simulink model "AERO560_HW1B_ThaparGagandeep"  (R2022b)
settings: Solver=VariableStepAuto  StartTime=0.0  StopTime=200.0  RelTol=1e-3
settings Model: Creator=gagandeepthapar  LastModifiedBy=gagandeepthapar

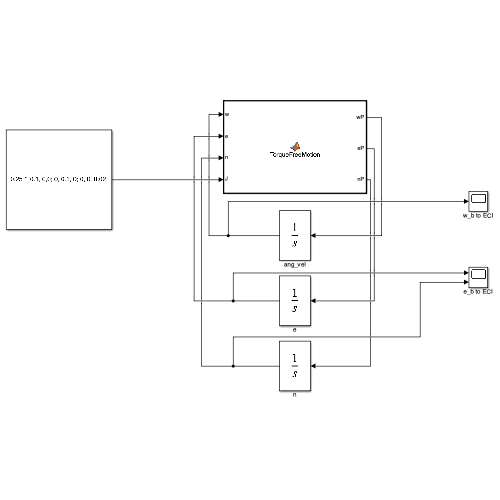
[thumbnail: Simulink's stored preview of the top-level diagram]
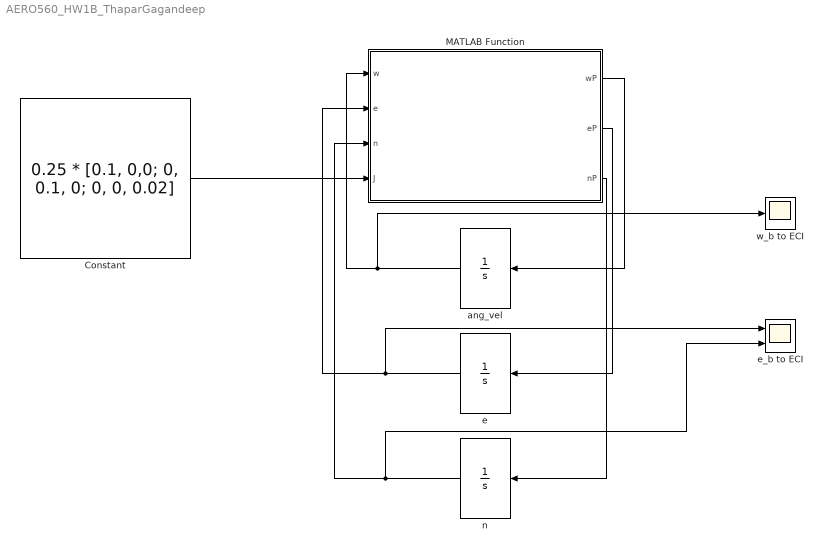
== system AERO560_HW1B_ThaparGagandeep ==
  Constant : Constant  Value=0.25 * [0.1, 0,0; 0, 0.1, 0; 0, 0, 0.02]
  MATLAB Function : MATLAB Function  TreatAsAtomicUnit=on
  ang_vel : Integrator  InitialCondition=[0.1; 0.1; 0.1]  ContinuousStateAttributes='ang_vel'
  e : Integrator  InitialCondition=[0;0;0]  ContinuousStateAttributes='e'
  e_b to ECI : Scope  NumInputPorts=2
  n : Integrator  InitialCondition=[1]  ContinuousStateAttributes='n'
  w_b to ECI : Scope
  wires:
  Constant/1 -> MATLAB Function/4(J)
  MATLAB Function/1(wP) -> ang_vel/1
  MATLAB Function/2(eP) -> e/1
  MATLAB Function/3(nP) -> n/1
  ang_vel/1 -> w_b to ECI/1, MATLAB Function/1(w)
  e/1 -> e_b to ECI/1, MATLAB Function/2(e)
  n/1 -> e_b to ECI/2, MATLAB Function/3(n)

== matlab function AERO560_HW1B_ThaparGagandeep/MATLAB Function ==
  data: w input; wP output; e input; n input; J input; eP output; nP output
function [wP, eP, nP] = TorqueFreeMotion(w,e,n, J)

    function wx = skewSymmetric(w)
        wx = [0, -1*w(3), w(2);
             w(3), 0, -1*w(1);
             -1*w(2), w(1), 0];
    end

    wP = -1*inv(J)*(skewSymmetric(w)*J*w);
    eP = 0.5*(n*ones(3) + skewSymmetric(e))*w;
    nP = -0.5*e'*w;

end
